simulink model "pam"  (R2018a)
settings: Solver=VariableStepAuto  StartTime=0.0  StopTime=2  RelTol=1e-3
libraries: dsparch4 x2, dspsigops x1
settings Model: Creator=hp  LastModifiedBy=hp

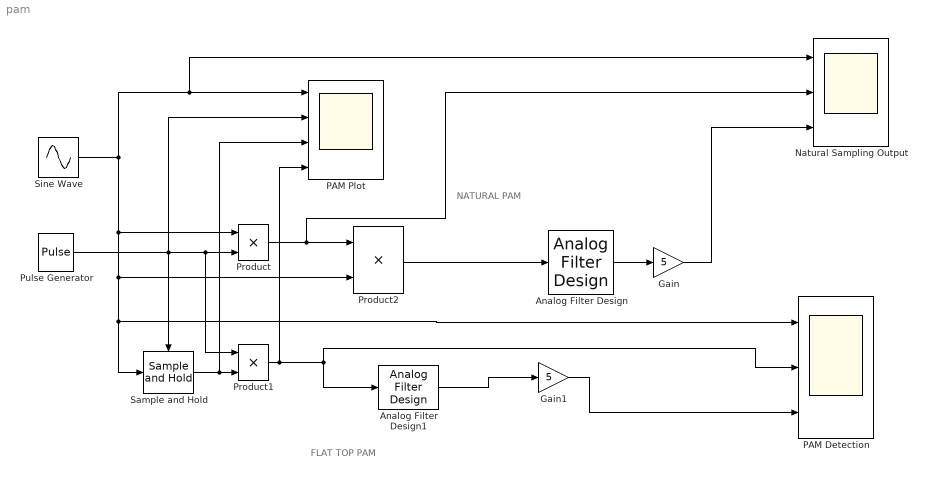
== system pam ==
  note: NATURAL PAM
  note: FLAT TOP PAM
  Analog Filter Design : dsparch4/Analog Filter Design  method=Butterworth  filttype=Lowpass  N=2  Wlo=2*pi*2  Whi=80  Rp=2  Rs=40
  Analog Filter Design1 : dsparch4/Analog Filter Design  method=Butterworth  filttype=Lowpass  N=2  Wlo=2*pi*2  Whi=80  Rp=2  Rs=40
  Gain : Gain  Gain=5
  Gain1 : Gain  Gain=5
  Natural Sampling Output : Scope  NumInputPorts=3
  PAM Detection : Scope  NumInputPorts=3
  "PAM Plot " : Scope  NumInputPorts=4
  Product : Product
  Product1 : Product
  Product2 : Product
  Pulse Generator : DiscretePulseGenerator  PulseType=Time based  Period=1/20  PulseWidth=25
  Sample and Hold : dspsigops/Sample and Hold  trig=Rising edge  initCond=0  latchinput=off
  Sine Wave : Sin  Frequency=2*pi*1  SampleTime=0
  wires:
  Pulse Generator/1 -> "PAM Plot "/2, Product1/1, Product/2, Sample and Hold/Trigger
  Sample and Hold/1 -> "PAM Plot "/3, Product1/2
  Product/1 -> Natural Sampling Output/2, Product2/1
  Product2/1 -> Analog Filter Design/1
  Sine Wave/1 -> Natural Sampling Output/1, "PAM Plot "/1, Product/1, PAM Detection/1, Sample and Hold/1, Product2/2
  Analog Filter Design/1 -> Gain/1
  Gain/1 -> Natural Sampling Output/3
  Product1/1 -> "PAM Plot "/4, PAM Detection/2, Analog Filter Design1/1
  Analog Filter Design1/1 -> Gain1/1
  Gain1/1 -> PAM Detection/3
